simulink model "HF_Backstepping_simulink"  (R2018b)
settings: Solver=VariableStepAuto  StartTime=0.0  StopTime=30  RelTol=1e-3
undefined symbols (not defined in the file): g, Iyy, l1, m
libraries: vrlib x3
settings Model: Creator=ferra  LastModifiedBy=ferra

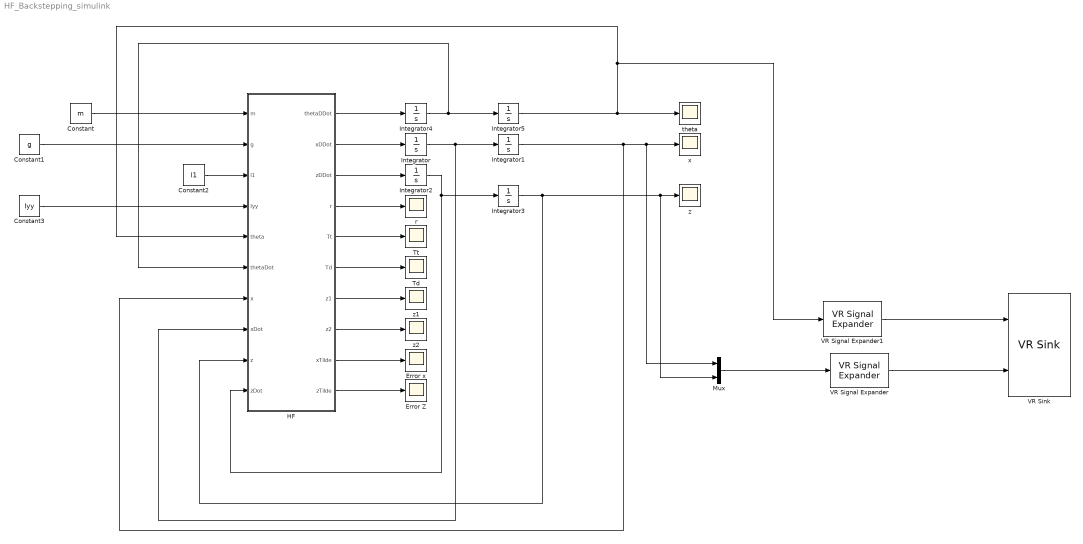
== system HF_Backstepping_simulink ==
  Constant : Constant  Value=m
  Constant1 : Constant  Value=g
  Constant2 : Constant  Value=l1
  Constant3 : Constant  Value=Iyy
  Error Z : Scope
  Error x : Scope
  "HF " : MATLAB Function  TreatAsAtomicUnit=on
  Integrator{,1..4} (5 alike) : Integrator
  Integrator5 : Integrator  InitialCondition=pi/8
  Mux : Mux  Inputs=2
  Td : Scope
  Tt : Scope
  VR Signal Expander : vrlib/VR Signal Expander  outwidth=3  outidx=[1 2]
      settings: SourceProductName=Simulink 3D Animation  SourceProductBaseCode=VR
  VR Signal Expander1 : vrlib/VR Signal Expander  outwidth=4  outidx=[4]
      settings: SourceProductName=Simulink 3D Animation  SourceProductBaseCode=VR
  VR Sink : vrlib/VR Sink  InstantiateOnLoad=on  SampleTime=0.3  ViewEnable=on  RemoteChange=off  RemoteView=off  FieldsWritten=Airplane.rotation.4.1.1.double#Airplane.translation.3.1.1.double  WorldFileName=C:\Users\ferra\Desktop\Projects\Matlab\Thesis\3D-simulation\3D_world.WRL  AutoView=off  VideoDimensions=[]  AllowVariableSize=off
      settings: SourceProductBaseCode=VR
  r : Scope
  theta : Scope
  x : Scope
  z : Scope
  z1 : Scope
  z2 : Scope
  wires:
  Integrator2/1 -> "HF "/10(zDot), Integrator3/1
  Constant3/1 -> "HF "/4(Iyy)
  Integrator/1 -> "HF "/8(xDot), Integrator1/1
  "HF "/3(zDDot) -> Integrator2/1
  "HF "/2(xDDot) -> Integrator/1
  Constant1/1 -> "HF "/2(g)
  "HF "/1(thetaDDot) -> Integrator4/1
  Constant2/1 -> "HF "/3(l1)
  Integrator4/1 -> Integrator5/1, "HF "/6(thetaDot)
  Integrator3/1 -> "HF "/9(z), Mux/2, z/1
  Integrator1/1 -> "HF "/7(x), Mux/1, x/1
  "HF "/4(r) -> r/1
  "HF "/6(Td) -> Td/1
  "HF "/5(Tt) -> Tt/1
  "HF "/7(z1) -> z1/1
  "HF "/8(z2) -> z2/1
  "HF "/9(xTilde) -> Error x/1
  "HF "/10(zTilde) -> Error Z/1
  Mux/1 -> VR Signal Expander/1
  VR Signal Expander1/1 -> VR Sink/1
  VR Signal Expander/1 -> VR Sink/2
  Integrator5/1 -> VR Signal Expander1/1, "HF "/5(theta), theta/1
  Constant/1 -> "HF "/1(m)

== matlab function HF_Backstepping_simulink/HF  ==
  data: thetaDDot output; m input; xDDot output; g input; l1 input; Iyy input; theta input; thetaDot input; x input; xDot input; z input; zDot input; zDDot output; r output; Tt output; Td output; z1 output; z2 output; xTilde output; zTilde output
function [thetaDDot,xDDot,zDDot, r, Tt,Td , z1,z2,xTilde,zTilde] = HF_dynamics(m,g,l1,Iyy,theta,thetaDot,x,xDot,z,zDot)

zDes = 5;
xDes = 3;

%saturation values
m1 = 0.9;
m2 = 2;
a = 1;
b = 2;
c= 1;

%gain of virutal controllers
kpz = 4;
kdz = 6;


k2 =  1;
k3 = 1;

%function between Td and thetaDot
g2 = -l1/Iyy;

%References
zTilde = z- zDes;
xTilde = x-xDes;


% %Control to stabilize z
r1 = sat(kpz*zTilde,m2) + kdz*zDot;
r = -sat(r1,m1);
Tt = (m*(g-r))/(cos(theta));

% %backstepping
phi1 =  sat(xTilde,a)+ sat(xDot,b);
z1 =phi1 - k2*theta;

% %z1Dot = satDot(x1Tilde,a)*xDot -k2*thetaDot + satDot(xDot,b)*(tan(theta)*(r-g));

% %Virtual Controller
n = -c*z1  - tan(theta)*satDot(xDot,b)*(r-g);
z2 = satDot(xTilde,a)*xDot - k2*thetaDot - n;

z1Dot = z2 - c*z1;

psi = satDot(xTilde,a)*tan(theta)*(r-g) ...
    + sec(theta)*sec(theta)*thetaDot*satDot(xDot,b)*(r-g)...
    +c*(z1Dot)+tan(theta)*satDot(xDot,b)*satDot(zTilde+zDot,m1)*(r-g);

%Controller 
Td = (psi + z1 + k3*z2)/(k2 * g2);

%Dynamics
xDDot = -Tt * sin(theta)/m;
zDDot = -Tt * cos(theta)/m + g;
thetaDDot = Td *g2;



end
